simulink model "Tut6_Switch_SwitchCase_Ifelse_"  (R2021a)
settings: Solver=VariableStepAuto  StartTime=0.0  StopTime=10.0  RelTol=1e-3
settings Model: Creator=cheta  LastModifiedBy=cheta

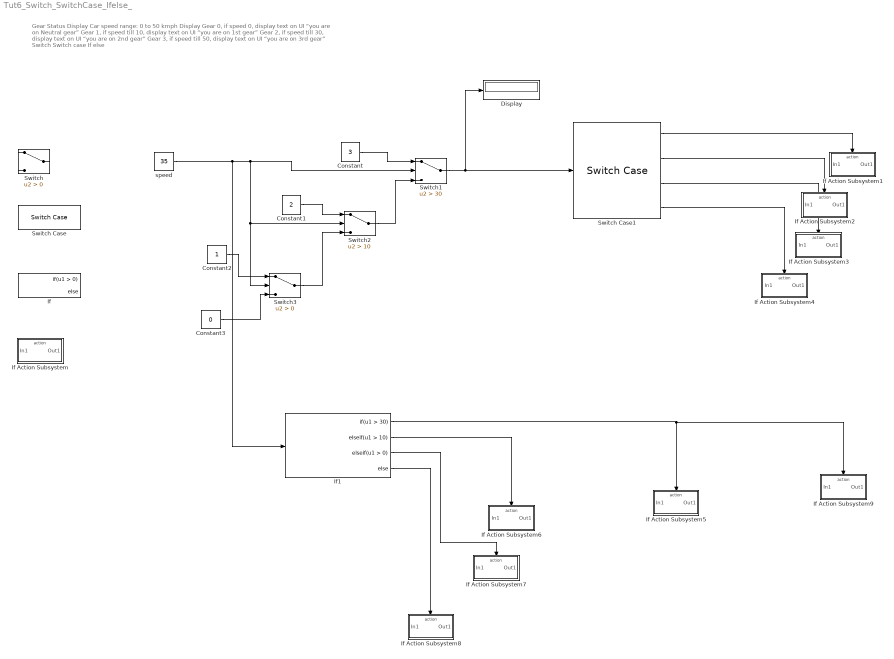
== system Tut6_Switch_SwitchCase_Ifelse_ ==
  note: Gear Status Display
      | Car speed range: 0 to 50 kmph
      | Display
      | Gear 0, if speed 0, display text on UI “you are on Neutral gear”
      | Gear 1, if speed till 10, display text on UI “you are on 1st gear”
      | Gear 2, if speed till 30, display text on UI “you are on 2nd gear”
      | Gear 3, if speed till 50, display text on UI “you are on 3rd gear”
      |
      | Switch
      | Switch case
      | If else
  Constant : Constant  Value=3
  Constant1 : Constant  Value=2
  Constant2 : Constant
  Constant3 : Constant  Value=0
  Display : Display
  If : If
  If Action Subsystem : Subsystem  TreatAsAtomicUnit=on
  If Action Subsystem1 : Subsystem  TreatAsAtomicUnit=on
  If Action Subsystem2 : Subsystem  TreatAsAtomicUnit=on
  If Action Subsystem3 : Subsystem  TreatAsAtomicUnit=on
  If Action Subsystem4 : Subsystem  TreatAsAtomicUnit=on
  If Action Subsystem5 : Subsystem  TreatAsAtomicUnit=on
  If Action Subsystem6 : Subsystem  TreatAsAtomicUnit=on
  If Action Subsystem7 : Subsystem  TreatAsAtomicUnit=on
  If Action Subsystem8 : Subsystem  TreatAsAtomicUnit=on
  If Action Subsystem9 : Subsystem  TreatAsAtomicUnit=on
  If1 : If  IfExpression=u1 > 30  ElseIfExpressions=u1 > 10, u1 > 0
  Switch : Switch  Criteria=u2 > Threshold
  Switch Case : SwitchCase
  Switch Case1 : SwitchCase  CaseConditions={3, 2, 1}
  Switch1 : Switch  Criteria=u2 > Threshold  Threshold=30
  Switch2 : Switch  Criteria=u2 > Threshold  Threshold=10
  Switch3 : Switch  Criteria=u2 > Threshold
  speed : Constant  Value=35
  wires:
  speed/1 -> If1/1, Switch3/2, Switch2/2, Switch1/2
  Constant/1 -> Switch1/1
  Constant1/1 -> Switch2/1
  Constant2/1 -> Switch3/1
  Constant3/1 -> Switch3/3
  Switch3/1 -> Switch2/3
  Switch2/1 -> Switch1/3
  Switch1/1 -> Display/1, Switch Case1/1
  Switch Case1/1 -> If Action Subsystem1/Action
  Switch Case1/2 -> If Action Subsystem2/Action
  Switch Case1/3 -> If Action Subsystem3/Action
  Switch Case1/4 -> If Action Subsystem4/Action
  If1/1 -> If Action Subsystem9/Action, If Action Subsystem5/Action
  If1/2 -> If Action Subsystem6/Action
  If1/3 -> If Action Subsystem7/Action
  If1/4 -> If Action Subsystem8/Action

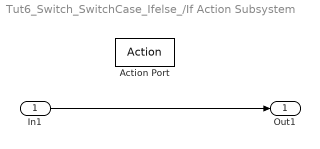
== system Tut6_Switch_SwitchCase_Ifelse_/If Action Subsystem ==
  In1 : Inport
  Action Port : ActionPort
  Out1 : Outport
  wires:
  In1/1 -> Out1/1

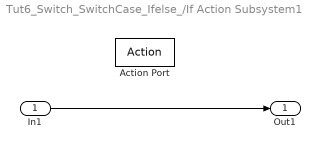
== system Tut6_Switch_SwitchCase_Ifelse_/If Action Subsystem1 ==
  In1 : Inport
  Action Port : ActionPort  ActionPortLabel=case [ 3 ]:
  Out1 : Outport
  wires:
  In1/1 -> Out1/1

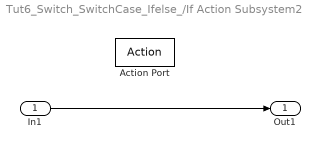
== system Tut6_Switch_SwitchCase_Ifelse_/If Action Subsystem2 ==
  In1 : Inport
  Action Port : ActionPort  ActionPortLabel=case [ 2 ]:
  Out1 : Outport
  wires:
  In1/1 -> Out1/1

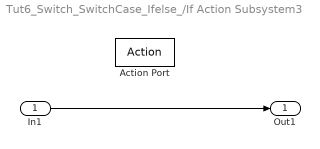
== system Tut6_Switch_SwitchCase_Ifelse_/If Action Subsystem3 ==
  In1 : Inport
  Action Port : ActionPort  ActionPortLabel=case [ 1 ]:
  Out1 : Outport
  wires:
  In1/1 -> Out1/1

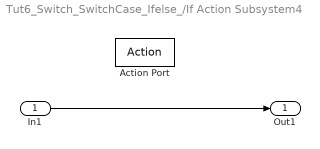
== system Tut6_Switch_SwitchCase_Ifelse_/If Action Subsystem4 ==
  In1 : Inport
  Action Port : ActionPort  ActionPortLabel=default:
  Out1 : Outport
  wires:
  In1/1 -> Out1/1

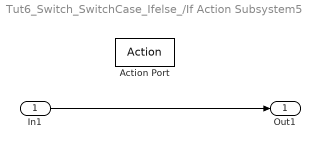
== system Tut6_Switch_SwitchCase_Ifelse_/If Action Subsystem5 ==
  In1 : Inport
  Action Port : ActionPort  ActionPortLabel=if(u1 > 30)
  Out1 : Outport
  wires:
  In1/1 -> Out1/1

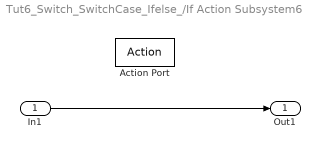
== system Tut6_Switch_SwitchCase_Ifelse_/If Action Subsystem6 ==
  In1 : Inport
  Action Port : ActionPort  ActionPortLabel=elseif(u1 > 10)
  Out1 : Outport
  wires:
  In1/1 -> Out1/1

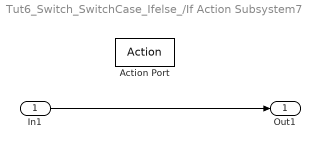
== system Tut6_Switch_SwitchCase_Ifelse_/If Action Subsystem7 ==
  In1 : Inport
  Action Port : ActionPort  ActionPortLabel=elseif( u1 > 0)
  Out1 : Outport
  wires:
  In1/1 -> Out1/1

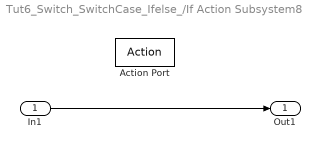
== system Tut6_Switch_SwitchCase_Ifelse_/If Action Subsystem8 ==
  In1 : Inport
  Action Port : ActionPort  ActionPortLabel=else
  Out1 : Outport
  wires:
  In1/1 -> Out1/1

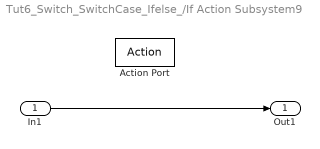
== system Tut6_Switch_SwitchCase_Ifelse_/If Action Subsystem9 ==
  In1 : Inport
  Action Port : ActionPort  ActionPortLabel=if(u1 > 30)
  Out1 : Outport
  wires:
  In1/1 -> Out1/1
